simulink model "TD1"  (R2017b)
settings: Solver=VariableStepAuto  StartTime=0.0  StopTime=0.2  RelTol=1e-3
InitFcn:
  | MCC_constants
StartFcn:
  | MCC_constants
undefined symbols (not defined in the file): b, J, K, L, R
settings Model: Creator=Table2  LastModifiedBy=Table2

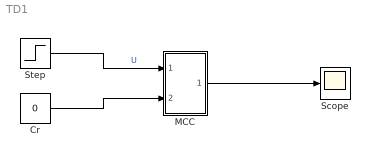
== system TD1 ==
  Cr : Constant  Value=0
  MCC : Subsystem
  Scope : Scope
  Step : Step  Time=0  After=12  SampleTime=0
  wires:
  Step/1 -> MCC/1(U Alim)  "U"
  Cr/1 -> MCC/2(C resist)
  MCC/1(Angle) -> Scope/1

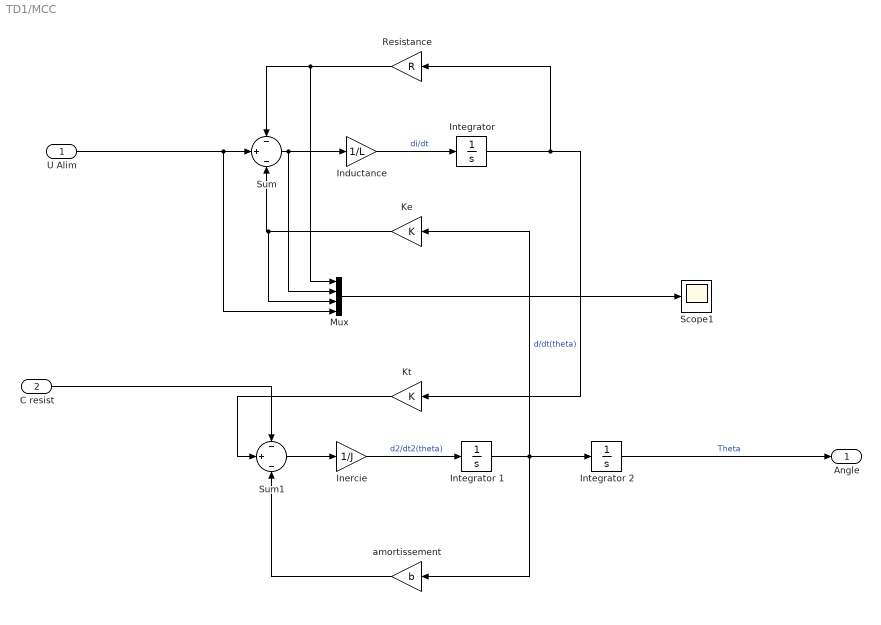
== system TD1/MCC ==
  U Alim : Inport
  C resist : Inport  Port=2
  Inductance : Gain  Gain=1/L
  Inercie : Gain  Gain=1/J
  "Integrator " : Integrator
  Integrator 1 : Integrator
  Integrator 2 : Integrator
  Ke : Gain  Gain=K
  Kt : Gain  Gain=K
  Mux : Mux
  Resistance : Gain  Gain=R
  Scope1 : Scope
  Sum : Sum  Inputs=-|+|-
  Sum1 : Sum  Inputs=-|+|-
  amortissement : Gain  Gain=b
  Angle : Outport
  wires:
  amortissement/1 -> Sum1/3
  Integrator 2/1 -> Angle/1  "Theta"
  Inercie/1 -> Integrator 1/1  "d2/dt2(theta)"
  U Alim/1 -> Mux/4, Sum/2
  Sum/1 -> Mux/2, Inductance/1
  C resist/1 -> Sum1/1
  Sum1/1 -> Inercie/1
  Resistance/1 -> Mux/1, Sum/1
  Mux/1 -> Scope1/1
  "Integrator "/1 -> Resistance/1, Kt/1
  Ke/1 -> Mux/3, Sum/3
  Kt/1 -> Sum1/2
  Integrator 1/1 -> Ke/1, amortissement/1, Integrator 2/1  "d/dt(theta)"
  Inductance/1 -> "Integrator "/1  "di/dt"
